simulink model "positioning_system_model"  (R2022b)
settings: Solver=VariableStepAuto  StartTime=0.0  StopTime=10.0  RelTol=1e-3
values from neighbouring files (symbols this model uses):
  C = 0.33 * 10^-6    (= 3.3e-07)    [run_positioning_system_model.m]
  d = 1    [run_positioning_system_model.m]
  km = 5 * 10^-3    (= 0.005)    [run_positioning_system_model.m]
  ks = 52.5    [run_positioning_system_model.m]
  P = 100 * 10^3    (= 100000)    [run_positioning_system_model.m]
  R = 10 * 10^3    (= 10000)    [run_positioning_system_model.m]
settings Model: Creator=royce  LastModifiedBy=royce

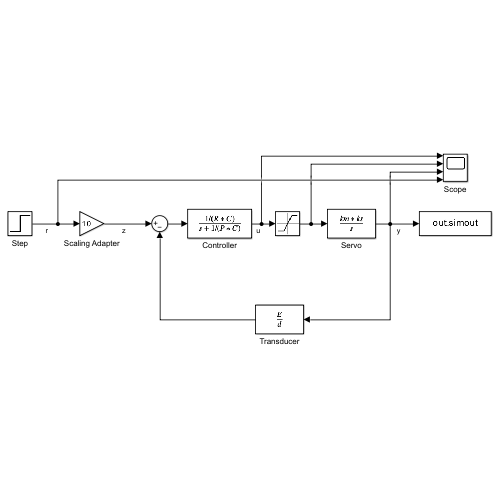
[thumbnail: Simulink's stored preview of the top-level diagram]
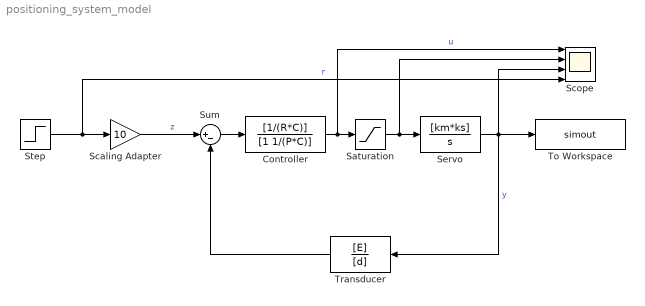
== system positioning_system_model ==
  Controller : TransferFcn  Numerator=[1/(R*C)]  Denominator=[1 1/(P*C)]  ParameterTunability=Unconstrained
  Saturation : Saturate  UpperLimit=100  LowerLimit=-10
  Scaling Adapter : Gain  Gain=10
  Scope : Scope  NumInputPorts=4
  Servo : TransferFcn  Numerator=[km*ks]  Denominator=[1 0]
  Step : Step  Time=3  After=0.5  SampleTime=0
  Sum : Sum  Inputs=|+-
  To Workspace : ToWorkspace  VariableName=simout  SaveFormat=Timeseries  SampleTime=-1
  Transducer : TransferFcn  Numerator=[E]  Denominator=[d]
  wires:
  Scaling Adapter/1 -> Sum/1  "z"
  Sum/1 -> Controller/1
  Controller/1 -> Scope/1, Saturation/1  "u"
  Servo/1 -> Scope/3, Transducer/1, To Workspace/1  "y"
  Transducer/1 -> Sum/2
  Step/1 -> Scope/4, Scaling Adapter/1  "r"
  Saturation/1 -> Scope/2, Servo/1
